simulink model "simulink_following_observer_R2020a"  (R2020a)
settings: Solver=ode4  StartTime=0.0  StopTime=15  FixedStep=0.01  RelTol=1e-3  EnableMultiTasking=on
values from neighbouring files (symbols this model uses):
  A = [  0      1      0      0 ... (first row only)    [following_observer.m]
  Av = [    0       1       0       0 ... (first row only)    [parameter_variation.m]
  B = [  0 ... (first row only)    [following_observer.m]
  Bv = [  0 ... (first row only)    [parameter_variation.m]
  C = [ 0  0  1  0 ]    [following_observer.m]
  H = [ -K  1 ]*inv(M0)*[ zeros(4,1) ... (first row only)    [following_observer.m]
  K = - acker(A,B,p)    [following_observer.m]
  L = - acker(A',C',q)'    [following_observer.m]
  x0 = [-0.5; 0; 0.5; 0]    [parameter_variation.m]
settings Model: Creator=kawata  LastModifiedBy=kawata
settings DataIOCC: LimitDataPoints=on  SaveFormat=Array  SignalLoggingSaveFormat=ModelDataLogs  ReturnWorkspaceOutputs=off
settings OptimizationCC: ExpressionDepthLimit=2147483647  LifeSpan=inf
settings DebuggingCC: UnderspecifiedInitializationDetection=Classic  MergeDetectMultiDrivingBlocksExec=none  SolverPrmCheckMsg=warning  FcnCallInpInsideContextMsg=warning  StateNameClashWarn=warning  SFUnexpectedBacktrackingDiag=warning  SFNoUnconditionalDefaultTransitionDiag=warning  SFExecutionAtInitializationDiag=none  ArithmeticOperatorsInVariantConditions=warning
settings HardwareCC: ProdBitPerPointer=32  ProdBitPerSizeT=32  ProdBitPerPtrDiffT=32  ProdLargestAtomicFloat=None  ProdIntDivRoundTo=Undefined  ProdEndianess=Unspecified  ProdWordSize=32  ProdHWDeviceType=32-bit Generic
settings ModelReferenceCC: PropagateSignalLabelsOutOfModel=off
settings SFSimCC: SimUseLocalCustomCode=off  CustomCodeUndefinedFunction=UseInterfaceOnly
settings RTWCC: RTWUseLocalCustomCode=off
settings CodeAppCC: StateflowObjectComments=on
settings GRTTargetCC: TargetLangStandard=C89/C90 (ANSI)  CombineOutputUpdateFcns=off  GRTInterface=on
settings ConfigComp: CovMetricSettings=dw  CovSaveCumulativeToWorkspaceVar=on  CovSaveSingleToWorkspaceVar=on  CovExternalEMLEnable=off

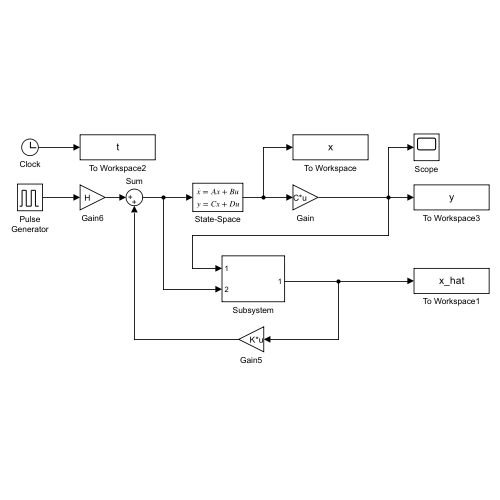
[thumbnail: Simulink's stored preview of the top-level diagram]
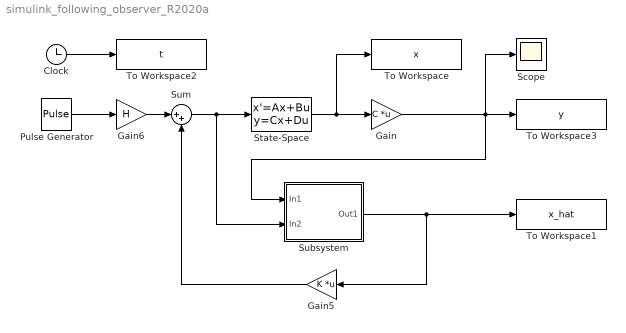
== system simulink_following_observer_R2020a ==
  Clock : Clock
  Gain : Gain  Gain=C  Multiplication=Matrix(K*u)
  Gain5 : Gain  Gain=K  Multiplication=Matrix(K*u)
  Gain6 : Gain  Gain=H
  Pulse Generator : DiscretePulseGenerator  PulseType=Time based  Period=10  PulseWidth=50
  Scope : Scope
  State-Space : StateSpace  A=Av  B=Bv  C=eye(4)  D=zeros(4,1)  InitialCondition=x0
  Subsystem : Subsystem
  Sum : Sum  Inputs=|++  InputSameDT=on  SaturateOnIntegerOverflow=on  OutDataTypeStr=Inherit: Same as first input
  To Workspace : ToWorkspace  VariableName=x  SampleTime=-1
  To Workspace1 : ToWorkspace  VariableName=x_hat  SampleTime=-1
  To Workspace2 : ToWorkspace  VariableName=t  SampleTime=-1
  To Workspace3 : ToWorkspace  VariableName=y  SampleTime=-1
  wires:
  State-Space/1 -> To Workspace/1, Gain/1
  Clock/1 -> To Workspace2/1
  Gain/1 -> To Workspace3/1, Subsystem/1(In1), Scope/1
  Pulse Generator/1 -> Gain6/1
  Gain6/1 -> Sum/1
  Sum/1 -> Subsystem/2(In2), State-Space/1
  Gain5/1 -> Sum/2
  Subsystem/1(Out1) -> To Workspace1/1, Gain5/1

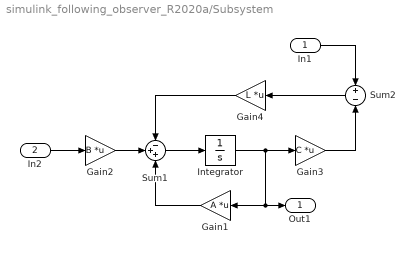
== system simulink_following_observer_R2020a/Subsystem ==
  In1 : Inport
  In2 : Inport  Port=2
  Gain1 : Gain  Gain=A  Multiplication=Matrix(K*u)  SaturateOnIntegerOverflow=on  OutDataTypeStr=Inherit: Same as input  ParamDataTypeStr=Inherit: Same as input
  Gain2 : Gain  Gain=B  Multiplication=Matrix(K*u)  SaturateOnIntegerOverflow=on  OutDataTypeStr=Inherit: Same as input  ParamDataTypeStr=Inherit: Same as input
  Gain3 : Gain  Gain=C  Multiplication=Matrix(K*u)  SaturateOnIntegerOverflow=on  OutDataTypeStr=Inherit: Same as input  ParamDataTypeStr=Inherit: Same as input
  Gain4 : Gain  Gain=L  Multiplication=Matrix(K*u)  SaturateOnIntegerOverflow=on  OutDataTypeStr=Inherit: Same as input  ParamDataTypeStr=Inherit: Same as input
  Integrator : Integrator
  Sum1 : Sum  Inputs=-++  InputSameDT=on  SaturateOnIntegerOverflow=on  OutDataTypeStr=Inherit: Same as first input
  Sum2 : Sum  Inputs=+|-  InputSameDT=on  SaturateOnIntegerOverflow=on  OutDataTypeStr=Inherit: Same as first input
  Out1 : Outport  VectorParamsAs1DForOutWhenUnconnected=off
  wires:
  In2/1 -> Gain2/1
  In1/1 -> Sum2/1
  Gain4/1 -> Sum1/1
  Sum2/1 -> Gain4/1
  Gain1/1 -> Sum1/3
  Gain2/1 -> Sum1/2
  Sum1/1 -> Integrator/1
  Integrator/1 -> Gain3/1, Out1/1, Gain1/1
  Gain3/1 -> Sum2/2
